simulink model "dp_kalman"  (R2015b)
settings: Solver=FixedStepAuto  StartTime=0.0  StopTime=5  FixedStep=T_s  RelTol=1e-3
InitFcn:
  | dp_kalman_script
values from neighbouring files (symbols this model uses):
  Ad = sysd.a    [dp_EKF_script.m]    (also in dp_kalman_script.m; dp_real_vs_lin_script.m; dp_statefeedback_script.m)
  Bd = sysd.b    [dp_EKF_script.m]    (also in dp_kalman_script.m; dp_real_vs_lin_script.m; dp_statefeedback_script.m)
  Cd_kalman = Cd(1,:)    [dp_kalman_script.m]    (also in dp_real_vs_lin_script.m)
  d_p1 = 0.001    [dp_EKF_script.m]    (also in dp_UKF_script.m; dp_kalman_script.m; dp_real_vs_lin_script.m; dp_statefeedback_script.m)
  d_p2 = 0.001    [dp_EKF_script.m]    (also in dp_UKF_script.m; dp_kalman_script.m; dp_real_vs_lin_script.m; dp_statefeedback_script.m)
  g = 9.81    [dp_EKF_script.m]    (also in dp_UKF_script.m; dp_kalman_script.m; dp_real_vs_lin_script.m; dp_statefeedback_script.m)
  l_1 = 0.194    [dp_EKF_script.m]    (also in dp_UKF_script.m; dp_kalman_script.m; dp_real_vs_lin_script.m; dp_statefeedback_script.m)
  l_2 = 0.1855    [dp_EKF_script.m]    (also in dp_UKF_script.m; dp_kalman_script.m; dp_real_vs_lin_script.m; dp_statefeedback_script.m)
  m_1 = 0.0313    [dp_EKF_script.m]    (also in dp_UKF_script.m; dp_kalman_script.m; dp_real_vs_lin_script.m; dp_statefeedback_script.m)
  m_2 = 0.0313    [dp_EKF_script.m]    (also in dp_UKF_script.m; dp_kalman_script.m; dp_real_vs_lin_script.m; dp_statefeedback_script.m)
  m_3 = 0.0308    [dp_EKF_script.m]    (also in dp_UKF_script.m; dp_kalman_script.m; dp_real_vs_lin_script.m; dp_statefeedback_script.m)
  Pk_0 = eye(4)    [dp_EKF_script.m]    (also in dp_UKF_script.m; dp_kalman_script.m = 1*eye(4); dp_real_vs_lin_script.m)
  Qk = zeros(4,4,steps,steps,steps,steps)    [dp_EKF_script.m]    (also in dp_UKF_script.m = zeros(4,4,9,9); dp_kalman_script.m = 1e-4*diag([1 1 1e-2 1e-2]); dp_real_vs_lin_script.m = 0*diag([1 1 1 1]))
  Rk = 1    [dp_EKF_script.m]    (also in dp_UKF_script.m; dp_kalman_script.m = 0.01; dp_real_vs_lin_script.m = 0.001)
  T_s = 0.001    [dp_EKF_script.m]    (also in dp_UKF_script.m; dp_kalman_script.m; dp_real_vs_lin_script.m; dp_statefeedback_script.m)
  x0 = [phi1_0; dphi1_0; phi2_0; dphi2_0]    [dp_EKF_script.m]    (also in dp_UKF_script.m; dp_kalman_script.m; dp_real_vs_lin_script.m; dp_statefeedback_script.m)
undefined symbols (not defined in the file or in its folder): K6_lqr
libraries: simulink x1
settings Model: Creator=serov  LastModifiedBy=serov

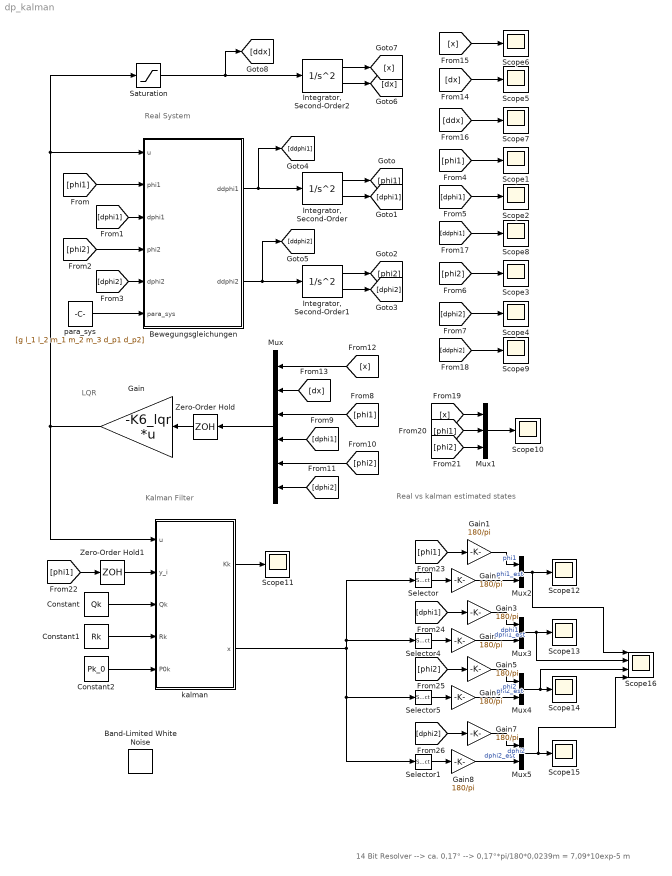
== system dp_kalman ==
  note: Real vs kalman estimated states
  note: LQR
  note: Real System
  note: Kalman Filter
  note: 14 Bit Resolver --> ca. 0,17° --> 0,17°*pi/180*0,0239m = 7,09*10exp-5 m
  Band-Limited White Noise : simulink/Sources/Band-Limited White Noise  Cov=0.5*0.000000003  Ts=0.001  seed=[23341]
  Bewegungsgleichungen : MATLAB Function  TreatAsAtomicUnit=on
  Constant : Constant  Value=Qk
  Constant1 : Constant  Value=Rk
  Constant2 : Constant  Value=Pk_0
  Gain : Gain  Gain=-K6_lqr  Multiplication=Matrix(K*u) (u vector)
  Gain{1..8} (8 alike) : Gain  Gain=180/pi
  "Integrator, Second-Order" : SecondOrderIntegrator  ICX=phi1_0  ICDXDT=dphi1_0
  "Integrator, Second-Order1" : SecondOrderIntegrator  ICX=phi2_0  ICDXDT=dphi2_0
  "Integrator, Second-Order2" : SecondOrderIntegrator  ICX=x_0  LimitX=on  UpperLimitX=0.2  LowerLimitX=-0.2  ICDXDT=dx_0  LimitDXDT=on  UpperLimitDXDT=5  LowerLimitDXDT=-5
  Mux : Mux  Inputs=6
  Mux1 : Mux  Inputs=3
  Mux{2..5} (4 alike) : Mux  Inputs=2
  Saturation : Saturate  UpperLimit=20  LowerLimit=-20
  Scope{1..15} (15 alike) : Scope
  Scope16 : Scope  NumInputPorts=4
  Selector : Selector  InputPortWidth=4  IndexOptions=Index vector (dialog)  Indices=[1]  OutputSizes=1
  Selector1 : Selector  InputPortWidth=4  IndexOptions=Index vector (dialog)  Indices=[4]  OutputSizes=1
  Selector4 : Selector  InputPortWidth=4  IndexOptions=Index vector (dialog)  Indices=[2]  OutputSizes=1
  Selector5 : Selector  InputPortWidth=4  IndexOptions=Index vector (dialog)  Indices=[3]  OutputSizes=1
  Zero-Order Hold : ZeroOrderHold  SampleTime=T_s
  Zero-Order Hold1 : ZeroOrderHold  SampleTime=T_s
  kalman : MATLAB Function  TreatAsAtomicUnit=on
  para_sys : Constant  Value=[g l_1 l_2 m_1 m_2 m_3 d_p1 d_p2]
  wires:
  Bewegungsgleichungen/1(ddphi1) -> [ddphi1], "Integrator, Second-Order"/1
  Bewegungsgleichungen/2(ddphi2) -> [ddphi2], "Integrator, Second-Order1"/1
  "Integrator, Second-Order"/1 -> [phi1]
  "Integrator, Second-Order"/2 -> [dphi1]
  "Integrator, Second-Order1"/2 -> [dphi2]
  "Integrator, Second-Order1"/1 -> [phi2]
  [phi1] -> Bewegungsgleichungen/2(phi1)
  [dphi1] -> Bewegungsgleichungen/3(dphi1)
  [phi2] -> Bewegungsgleichungen/4(phi2)
  [dphi2] -> Bewegungsgleichungen/5(dphi2)
  para_sys/1 -> Bewegungsgleichungen/6(para_sys)
  [phi1] -> Scope1/1
  [dphi1] -> Scope2/1
  [phi2] -> Scope3/1
  [dphi2] -> Scope4/1
  [phi1] -> Mux/3
  [dphi1] -> Mux/4
  [phi2] -> Mux/5
  [dphi2] -> Mux/6
  Mux/1 -> Zero-Order Hold/1
  "Integrator, Second-Order2"/1 -> [x]
  "Integrator, Second-Order2"/2 -> [dx]
  [x] -> Mux/1
  [dx] -> Mux/2
  Gain/1 -> kalman/1(u), Saturation/1, Bewegungsgleichungen/1(u)
  [dx] -> Scope5/1
  [x] -> Scope6/1
  [ddx] -> Scope7/1
  [ddphi1] -> Scope8/1
  [ddphi2] -> Scope9/1
  Saturation/1 -> [ddx], "Integrator, Second-Order2"/1
  Mux1/1 -> Scope10/1
  [x] -> Mux1/1
  [phi1] -> Mux1/2
  [phi2] -> Mux1/3
  Constant/1 -> kalman/3(Qk)
  Constant1/1 -> kalman/4(Rk)
  Constant2/1 -> kalman/5(P0k)
  [phi1] -> Zero-Order Hold1/1
  kalman/1(Kk) -> Scope11/1
  kalman/2(x) -> Selector/1, Selector4/1, Selector1/1, Selector5/1
  Zero-Order Hold/1 -> Gain/1
  Selector/1 -> Gain2/1
  Gain2/1 -> Mux2/2  "phi1_est"
  Mux2/1 -> Scope16/1, Scope12/1
  [phi1] -> Gain1/1
  Gain1/1 -> Mux2/1  "phi1"
  Selector4/1 -> Gain4/1
  Gain4/1 -> Mux3/2  "dphi1_est"
  Mux3/1 -> Scope16/2, Scope13/1
  [dphi1] -> Gain3/1
  Gain3/1 -> Mux3/1  "dphi1"
  Selector5/1 -> Gain6/1
  Gain6/1 -> Mux4/2  "phi2_est"
  Mux4/1 -> Scope16/3, Scope14/1
  [phi2] -> Gain5/1
  Gain5/1 -> Mux4/1  "phi2"
  Selector1/1 -> Gain8/1
  Gain8/1 -> Mux5/2  "dphi2_est"
  Mux5/1 -> Scope16/4, Scope15/1
  [dphi2] -> Gain7/1
  Gain7/1 -> Mux5/1  "dphi2"
  Zero-Order Hold1/1 -> kalman/2(y_i)

== matlab function dp_kalman/kalman ==
  data: u input; y_i input; Qk input size=[4 4]; Rk input; Ad parameter; Bd parameter; Cd_kalman parameter; Kk output size=[4 1]; x output size=[4 1]; x0 parameter; P0k input
function [Kk, x] = fcn(u, y_i, Qk, Rk, Ad, Bd, Cd_kalman, x0, P0k)
%#codegen
persistent x_p P_p
%% Initialisierung im ersten Zeitschritt wird nur einmal aufgerufen
if isempty(x_p)
    x_p = zeros(4,1);
    x = zeros(4,1);
% korrekte Initialisierung
%    x_p = x0;    
%    x = x_p;
    P_p = P0k;
    Kk = zeros(4,1); 
else
%% Discrete Time update: prediction
x = Ad*x_p + Bd * u;
P = Ad*P_p*Ad' + Qk;
%% Measurement update: correction
Kk = P*Cd_kalman' *(Cd_kalman*P*Cd_kalman' + Rk)^(-1);
x = x + Kk * (y_i - Cd_kalman*x);
P = (eye(4) - Kk *Cd_kalman)*P;
x_p = x;
P_p = P;
end

== matlab function dp_kalman/Bewegungsgleichungen ==
  data: u input; phi1 input; dphi1 input; phi2 input; dphi2 input; para_sys input; ddphi1 output; ddphi2 output
function [ddphi1, ddphi2] = pendel_1_2(u, phi1, dphi1, phi2, dphi2, para_sys)
%#codegen

g = para_sys(1);
l_1 = para_sys(2);
l_2 = para_sys(3);
m_1 = para_sys(4);
m_2 = para_sys(5);
m_3 = para_sys(6);
d_p1 = para_sys(7);
d_p2 = para_sys(8);

ddphi1 = 1/(l_1^2*(9*cos(phi1-phi2)^2*m_2-4*m_1-12*m_2-12*m_3)*l_2)*(9*dphi1^2*cos(phi1-phi2)*sin(phi1-phi2)*l_1^2*l_2*m_2+6*m_2*l_1*l_2^2*sin(phi1-phi2)*dphi2^2+9*u*cos(phi1-phi2)*cos(phi2)*l_1*l_2*m_2+9*cos(phi1-phi2)*sin(phi2)*g*l_1*l_2*m_2-6*l_1*cos(phi1)*u*m_1*l_2-12*l_1*cos(phi1)*u*m_2*l_2-12*l_1*cos(phi1)*u*m_3*l_2-6*l_1*g*sin(phi1)*m_1*l_2-12*l_1*g*sin(phi1)*m_2*l_2-12*l_1*g*sin(phi1)*m_3*l_2+18*dphi1*cos(phi1-phi2)*d_p2*l_1-18*dphi2*cos(phi1-phi2)*d_p2*l_1+12*dphi1*d_p1*l_2+12*dphi1*d_p2*l_2-12*d_p2*dphi2*l_2);

ddphi2 = -1/(l_1*l_2^2*(9*cos(phi1-phi2)^2*m_2-4*m_1-12*m_2-12*m_3)*m_2)*(12*dphi1*d_p2*l_1*m_1+36*dphi1*d_p2*l_1*m_2+36*dphi1*d_p2*l_1*m_3-12*dphi2*d_p2*l_1*m_1-36*dphi2*d_p2*l_1*m_2-36*dphi2*d_p2*l_1*m_3-9*cos(phi1)*u*cos(phi1-phi2)*l_1*l_2*m_1*m_2-18*cos(phi1)*u*cos(phi1-phi2)*l_1*l_2*m_2*m_3-9*cos(phi1-phi2)*sin(phi1)*g*l_1*l_2*m_1*m_2-18*cos(phi1-phi2)*sin(phi1)*g*l_1*l_2*m_2*m_3+9*dphi2^2*cos(phi1-phi2)*sin(phi1-phi2)*l_1*l_2^2*m_2^2+ 6*dphi1^2*sin(phi1-phi2)*l_1^2*l_2*m_1*m_2+ 18*dphi1^2*sin(phi1-phi2)*l_1^2*l_2*m_2*m_3-18*cos(phi1)*u*cos(phi1-phi2)*l_1*l_2*m_2^2-18*cos(phi1-phi2)*sin(phi1)*g*l_1*l_2*m_2^2 +6*u*cos(phi2)*l_1*l_2*m_1*m_2+18*u*cos(phi2)*l_1*l_2*m_2*m_3+6*sin(phi2)*g*l_1*l_2*m_1*m_2+18*sin(phi2)*g*l_1*l_2*m_2*m_3 + 18*(dphi1)^2*sin(phi1-phi2)*l_1^2*l_2*m_2^2+18*u*cos(phi2)*l_1*l_2*m_2^2+18*sin(phi2)*g*l_1*l_2*m_2^2+18*dphi1*cos(phi1-phi2)*d_p1*l_2*m_2 + 18*dphi1*cos(phi1-phi2)*d_p2*l_2*m_2-18*dphi2*cos(phi1-phi2)*d_p2*l_2*m_2);
